simulink model "controller_blockDiagram"  (R2015b)
settings: Solver=VariableStepAuto  StartTime=0.0  StopTime=10.0  RelTol=1e-3
undefined symbols (not defined in the file): Kd, Kff, Ki, Kp
settings Model: Creator=DC  LastModifiedBy=DC

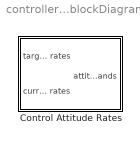
== system controller_blockDiagram ==
  Control Attitude Rates : Subsystem

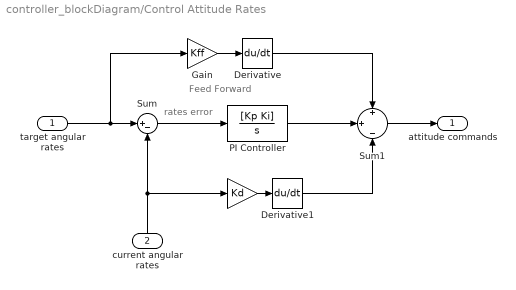
== system controller_blockDiagram/Control Attitude Rates ==
  note: rates error
  note: Feed Forward
  target angular rates : Inport
  current angular rates : Inport  Port=2
  " " : Gain  Gain=Kd
  Derivative : Derivative
  Derivative1 : Derivative
  Gain : Gain  Gain=Kff
  PI Controller : TransferFcn  Numerator=[Kp Ki]  Denominator=[1 0]
  Sum : Sum  Inputs=|+-
  Sum1 : Sum  Inputs=+|+|-
  attitude commands : Outport
  wires:
  Derivative1/1 -> Sum1/3
  target angular rates/1 -> Gain/1, Sum/1
  PI Controller/1 -> Sum1/2
  current angular rates/1 -> " "/1, Sum/2
  Sum/1 -> PI Controller/1
  Derivative/1 -> Sum1/1
  Gain/1 -> Derivative/1
  " "/1 -> Derivative1/1
  Sum1/1 -> attitude commands/1
